simulink model "BasePerTracing"  (R2024b)
settings: Solver=FixedStepDiscrete  StartTime=0.0  StopTime=Inf  RelTol=1e-3  EnableMultiTasking=on
InitFcn:
  | mcb_pmsm_foc_qep_f28379d_data;
values from neighbouring files (symbols this model uses):
  ADCCount = ADCResolution-1    (= 4095)    [BaseModelForControl_Parameters.m]    (also in dc_motor_data.m)
  Dz_dahlin = minreal(Dz_dahlin)    [dc_motor_data.m]
  Dz_deadbeat = (1/Gpz)*((z^-k)/(1-(z^-k)))    [dc_motor_data.m]
  GainVsense = 4.99/(62+4.99)    (= 0.0744887296611)    [BaseModelForControl_Parameters.m]    (also in dc_motor_data.m)
  GammaZ = 40*(z-0.8)*(z-0.9)*(z-0.7)    [DeadBeatModel_Parameters_Student.m]    (also in dc_motor_data.m)
  J = 0.352e-4    (= 3.52e-05)    [DC_MotorEquation_Encoder_Parameters.m]    (also in DahlinModel_Parameters_Student.m = 7.32e-05; DeadBeatModel_Parameters_Student.m = 0.00010043; dc_motor_data.m = 0.00010043)
  Km = 0.11    [DC_MotorEquation_Encoder_Parameters.m]    (also in DahlinModel_Parameters_Student.m; DeadBeatModel_Parameters_Student.m; dc_motor_data.m)
  Kpi = L/tao_pid_current    (= 6.2)    [dc_motor_data.m]
  Kpw = J/(tao_pid_speed*Km)    (= 0.0913)    [dc_motor_data.m]
  OffsetADCINC4 = 2296    [BaseModelForControl_Parameters.m]    (also in dc_motor_data.m)
  PulseNumber = 2048*4    (= 8192)    [BaseModelForControl_Parameters.m]    (also in DC_MotorEquation_Encoder_Parameters.m; DahlinModel_Parameters_Student.m; DeadBeatModel_Parameters_Student.m; dc_motor_data.m)
  RadiantsPerCount = 2*pi/(PulseNumber-1)    (= 0.00076708403213)    [BaseModelForControl_Parameters.m]    (also in DC_MotorEquation_Encoder_Parameters.m; DahlinModel_Parameters_Student.m; DeadBeatModel_Parameters_Student.m; dc_motor_data.m)
  RpmToRads = 2*pi/60    (= 0.10471975512)    [BaseModelForControl_Parameters.m]    (also in DC_MotorEquation_Encoder_Parameters.m; DahlinModel_Parameters_Student.m; DeadBeatModel_Parameters_Student.m; dc_motor_data.m)
  TaoFilterOffsetCurrent = 1    [BaseModelForControl_Parameters.m]    (also in dc_motor_data.m)
  TaoFilterOmega = b_filter*TSample/a_filter    (= 0.0009)    [BaseModelForControl_Parameters.m]    (also in DahlinModel_Parameters_Student.m = 0.002; DeadBeatModel_Parameters_Student.m = 0.005; dc_motor_data.m = 0.005)
  Tii = L/R    (= 0.00190505453987)    [dc_motor_data.m]
  Tiw = tao_m    (= 0.0913)    [dc_motor_data.m]
  TSample = PWM_Period    (= 0.0001)    [BaseModelForControl_Parameters.m]    (also in DahlinModel_Parameters_Student.m; DeadBeatModel_Parameters_Student.m; dc_motor_data.m)
  VrefADC = 3    [BaseModelForControl_Parameters.m]    (also in dc_motor_data.m)
undefined symbols (not defined in the file or in its folder): dataType, Down, dspblkCoreblockFVToolHelper, gcbh, GPTRIP1SEL, GPTRIP2SEL, TZ1, TZ2, Up
libraries: c2802xlib x9, simulink x8, c280xlib x4, c2837xDlib x3, c2000lib x1, svdutilitieslib x1
(part 2 of 2)

== system BasePerTracing/Current Control/SCI (Code Generation)/While Iterator Subsystem ==
  Data : Inport
  Iteration : Inport  Port=2
  Add : Sum  Inputs=+-  OutDataTypeStr=Inherit: Same as first input
  Index Vector : MultiPortSwitch  Inputs=1  SaturateOnIntegerOverflow=off  InputSameDT=off
  SCI Transmit : c280xlib/SCI Transmit  sciModule=A  dataHead=''  dataTail=''  frameSize=1  blockingMode=on  outputStatus=off
  While Iterator : WhileIterator  MaxIters=-1  WhileBlockType=do-while  ShowIterationPort=on  OutputDataType=int16
  wires:
  While Iterator/1 -> Add/2, Index Vector/1
  Data/1 -> Index Vector/2
  Index Vector/1 -> SCI Transmit/1
  Add/1 -> While Iterator/1
  Iteration/1 -> Add/1

== system BasePerTracing/Serial Receive/Code Generation/Data_Type_Fixed_Point ==
  SCI Receive : c280xlib/SCI Receive  sciModule=A  dataHead=''  headerCheckMaxCount=16  dataTail=''  dataType=uint32  dataLenOptions=Length via dialog  dataDim=2  maxDataLength=1  initValue=0  errOption=Output the last received value  errValue=0  sampleTime=-1  blockingMode=on  timeOut=0.00875  outputStatus=off
  Out1 : Outport
  wires:
  SCI Receive/1 -> Out1/1

== system BasePerTracing/Serial Receive/Code Generation/Data_Type_Float ==
  SCI Receive : c280xlib/SCI Receive  sciModule=A  dataHead=''  headerCheckMaxCount=16  dataTail=''  dataType=single  dataLenOptions=Length via dialog  dataDim=2  maxDataLength=1  initValue=0  errOption=Output the last received value  errValue=0  sampleTime=-1  blockingMode=on  timeOut=0.00875  outputStatus=off
  Out1 : Outport
  wires:
  SCI Receive/1 -> Out1/1

== system BasePerTracing/Serial Receive/Data_Conditioning_Rx/Data_Type_Fixed_Point ==
  In1 : Inport
  Data Type Conversion1 : DataTypeConversion  OutDataTypeStr=dataType  RndMeth=Simplest  SaturateOnIntegerOverflow=off
  Data Type Conversion2 : DataTypeConversion  OutDataTypeStr=fixdt(1,32,28)  ConvertRealWorld=Stored Integer (SI)  RndMeth=Simplest  SaturateOnIntegerOverflow=off
  Data Type Conversion3 : DataTypeConversion  OutDataTypeStr=uint16  RndMeth=Simplest  SaturateOnIntegerOverflow=off
  Demux : Demux  Outputs=2
  Desired Speed : Outport
  Out2 : Outport  Port=2
  wires:
  In1/1 -> Demux/1
  Data Type Conversion1/1 -> Desired Speed/1
  Data Type Conversion2/1 -> Data Type Conversion1/1
  Demux/1 -> Data Type Conversion2/1
  Demux/2 -> Data Type Conversion3/1
  Data Type Conversion3/1 -> Out2/1

== system BasePerTracing/Serial Receive/Data_Conditioning_Rx/Data_Type_Float ==
  In1 : Inport
  Data Type Conversion2 : DataTypeConversion  OutDataTypeStr=uint16  RndMeth=Simplest  SaturateOnIntegerOverflow=off
  Demux : Demux  Outputs=2
  Desired Speed : Outport
  Out2 : Outport  Port=2
  wires:
  In1/1 -> Demux/1
  Demux/1 -> Desired Speed/1
  Data Type Conversion2/1 -> Out2/1
  Demux/2 -> Data Type Conversion2/1

== system BasePerTracing/Current Control/SCI (Code Generation)/Data_Conditioning_Tx/Data_Type_Fixed_Point ==
  In1 : Inport
  Data Type Conversion : DataTypeConversion  OutDataTypeStr=fixdt(1,32,28)  RndMeth=Simplest  SaturateOnIntegerOverflow=off
  Data Type Conversion3 : DataTypeConversion  OutDataTypeStr=uint32  ConvertRealWorld=Stored Integer (SI)  RndMeth=Simplest  SaturateOnIntegerOverflow=off
  Data_Log : Outport
  wires:
  In1/1 -> Data Type Conversion/1
  Data Type Conversion3/1 -> Data_Log/1
  Data Type Conversion/1 -> Data Type Conversion3/1

== system BasePerTracing/Current Control/SCI (Code Generation)/Data_Conditioning_Tx/Data_Type_Float ==
  In1 : Inport
  Byte Pack : svdutilitieslib/Byte Pack  maskPackedDataType=uint32  datatypes={'single'}  byteAlign=4  blockPlatform=tic2000
  Data_Log : Outport
  wires:
  Byte Pack/1 -> Data_Log/1
  In1/1 -> Byte Pack/1

== system BasePerTracing/Current Control/SCI (Code Generation)/Data_Logging/Data ==
  Data : Inport
  Data_width : Inport  Port=2
  Action Port : ActionPort  ActionPortLabel=else
  Dummy : Constant  Value=hex2dec('0000')  OutDataTypeStr=uint32
  Mux : Mux  Inputs=2
  Data_out : Outport  VectorParamsAs1DForOutWhenUnconnected=off
  Iteration : Outport  Port=2  VectorParamsAs1DForOutWhenUnconnected=off
  wires:
  Data_width/1 -> Iteration/1
  Data/1 -> Mux/1
  Dummy/1 -> Mux/2
  Mux/1 -> Data_out/1

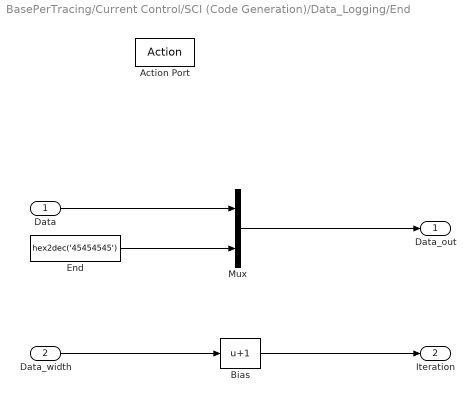
== system BasePerTracing/Current Control/SCI (Code Generation)/Data_Logging/End ==
  Data : Inport
  Data_width : Inport  Port=2
  Action Port : ActionPort  ActionPortLabel=elseif(u1 == 599)
  Bias : Bias  Bias=1  SaturateOnIntegerOverflow=off
  End : Constant  Value=hex2dec('45454545')  OutDataTypeStr=uint32
  Mux : Mux  Inputs=2
  Data_out : Outport  VectorParamsAs1DForOutWhenUnconnected=off
  Iteration : Outport  Port=2  VectorParamsAs1DForOutWhenUnconnected=off
  wires:
  Data/1 -> Mux/1
  Data_width/1 -> Bias/1
  Bias/1 -> Iteration/1
  End/1 -> Mux/2
  Mux/1 -> Data_out/1

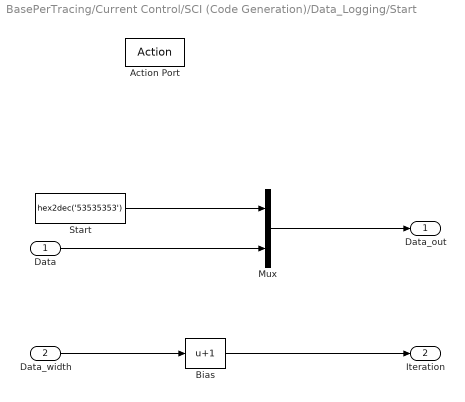
== system BasePerTracing/Current Control/SCI (Code Generation)/Data_Logging/Start ==
  Data : Inport
  Data_width : Inport  Port=2
  Action Port : ActionPort  ActionPortLabel=if(u1 == 0)
  Bias : Bias  Bias=1  SaturateOnIntegerOverflow=off
  Mux : Mux  Inputs=2
  Start : Constant  Value=hex2dec('53535353')  OutDataTypeStr=uint32
  Data_out : Outport  VectorParamsAs1DForOutWhenUnconnected=off
  Iteration : Outport  Port=2  VectorParamsAs1DForOutWhenUnconnected=off
  wires:
  Data/1 -> Mux/2
  Data_width/1 -> Bias/1
  Bias/1 -> Iteration/1
  Start/1 -> Mux/1
  Mux/1 -> Data_out/1

== matlab function BasePerTracing/Current Control/AnalogReading/MATLAB Function ==
  data: Ts input; out output; Tao input; In input
function out  = LowPassFilter(  Ts ,Tao, In)

persistent OutPrecedente
if isempty( OutPrecedente )
    OutPrecedente = 0 ;
end
    %Filtro passa basso discretizzato con il metodo delle differenze
    %all'indietro
    
    a=Ts/(Ts+Tao);
    b=Tao/(Ts+Tao);
    
    out=a*In+OutPrecedente*b;
   
    OutPrecedente = out;
   
end

== matlab function BasePerTracing/Current Control/ENCODER/MATLAB Function1 ==
  data: Ts input; ThetaMis output; RadiantiPerCount input; Counter input; OmegaMis output; OmegaMisRPM output; DeltaCounter output
function [ThetaMis, OmegaMis, OmegaMisRPM, DeltaCounter] = CounterToThetaOmega(Ts, RadiantiPerCount, Counter)

% Inizializzazione dei valori iniziali 
persistent CounterPrec  
if isempty( CounterPrec )
    CounterPrec = 0;
end 

    DeltaCounter=Counter-CounterPrec;
    
    if (DeltaCounter>double(0x1000))
        DeltaCounter=DeltaCounter-double(0x2000);
    end
    
    if (DeltaCounter<-double(0x1000))
        DeltaCounter=DeltaCounter+double(0x2000);
    end
        
    % conversione conteggio in radianti
    ThetaMis = Counter * RadiantiPerCount;
    
    DeltaThetaMis = DeltaCounter*RadiantiPerCount;
   
    OmegaMis = DeltaThetaMis/Ts;
    OmegaMisRPM=OmegaMis*60/(2*pi);
 
    CounterPrec= Counter;
end

== matlab function BasePerTracing/Current Control/ENCODER/MATLAB Function ==
  data: Ts input; out output; Tao input; In input
function out = LowPassFilter( Ts ,Tao, In)
persistent OutPrecedente
if isempty( OutPrecedente )
 OutPrecedente = 0 ;
end
% Filtro passa basso discretizzato con il
 % metodo delle differenze all'indietro

 a=Ts/(Ts+Tao);
 b=Tao/(Ts+Tao);

 out=a*In+OutPrecedente*b;

 OutPrecedente = out;

end

== matlab function BasePerTracing/Current Control/MATLAB Function1 ==
  settings: updateMethod=DISCRETE
  data: in input; out output; Kp input; Ti input; Ts input; Enable input; EnableCheckSat input; HiSat input; LowSat input; omega_m input
function out = PI( in ,Kp , Ti , Ts , Enable, EnableCheckSat, HiSat, LowSat, omega_m)
persistent in_prev out_prev
% Initial Value
if isempty( out_prev )
out_prev = 0;
end
if isempty( in_prev )
in_prev = 0;
end

% G(s)=(Kp/Ti)*((1+Ti*s)/s) (Tustin)
% We run control only if motor is running
if (Enable == 1)
%I Calculate the output
 out = Kp*Ts/(2*Ti)*(in+in_prev) + Kp*(in-in_prev) + out_prev ;
else
out = 0;
in = 0;
end

if(EnableCheckSat == 1)
%check for saturation
if out > HiSat
out = HiSat;
elseif (out < LowSat)
out = LowSat;
end
end

out_prev = out;
in_prev = in;
end

== matlab function BasePerTracing/Current Control/MATLAB Function2 ==
  settings: updateMethod=DISCRETE
  data: in input; out output; Kp input; Ti input; Ts input; Enable input; EnableCheckSat input; HiSat input; LowSat input; omega_m input
function out = PI( in ,Kp , Ti , Ts , Enable, EnableCheckSat, HiSat, LowSat, omega_m)
persistent in_prev out_prev
% Initial Value
if isempty( out_prev )
out_prev = 0;
end
if isempty( in_prev )
in_prev = 0;
end

% G(s)=(Kp/Ti)*((1+Ti*s)/s) (Tustin)
% We run control only if motor is running
if (Enable == 1)
%I Calculate the output
 out = Kp*Ts/(2*Ti)*(in+in_prev) + Kp*(in-in_prev) + out_prev ;
else
out = 0;
in = 0;
end

if(EnableCheckSat == 1)
%check for saturation
if out > HiSat
out = HiSat;
elseif (out < LowSat)
out = LowSat;
end
end

out_prev = out;
in_prev = in;
end
